simulink model "Controller_Algorithm_Local"  (R2025b)
settings: Solver=FixedStepAuto  StartTime=0.0  StopTime=10.0  RelTol=1e-3
InitFcn:
  | Simulink.defineIntEnumType(...
  | 'modeSchedulerEnum', ...
  | {'Error', 'OpenLoopVelocity', 'CalibrateEncoder', 'Velocity'}, ...
  | [0, 1, 2, 3]);
values from neighbouring files (symbols this model uses):
  sampleTime = 4.0E-5    [FoCFpgaData.sldd]
settings Model: DataDictionary=FoCFpgaData.sldd  Creator=Admin  LastModifiedBy=Admin
settings SolverCC: ZeroCrossAlgorithm=Adaptive
settings DataIOCC: LimitDataPoints=on  SaveFormat=Structure  SaveOutput=off  SaveTime=off
settings OptimizationCC: DefaultParameterBehavior=Inlined  UseDivisionForNetSlopeComputation=on
settings ConfigComp: CovMetricSettings=dw  CovSaveCumulativeToWorkspaceVar=on  CovSaveSingleToWorkspaceVar=on  CovExternalEMLEnable=off  CovSFcnEnable=off

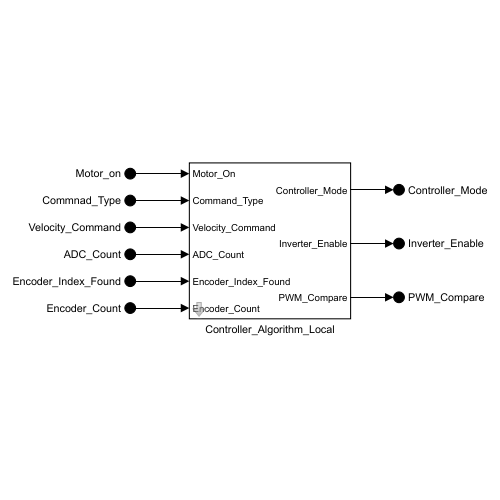
[thumbnail: Simulink's stored preview of the top-level diagram]
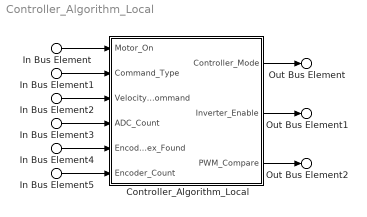
== system Controller_Algorithm_Local ==
  In Bus Element : Inport  PortName=Motor_on
  In Bus Element1 : Inport  Port=2  PortName=Commnad_Type
  In Bus Element2 : Inport  Port=3  PortName=Velocity_Command
  In Bus Element3 : Inport  Port=4  PortName=ADC_Count
  In Bus Element4 : Inport  Port=5  PortName=Encoder_Index_Found
  In Bus Element5 : Inport  Port=6  PortName=Encoder_Count
  Controller_Algorithm_Local : Subsystem
      mask help: Simulink:masks:GenSFuncDesc_MD
      mask Help: eval('feval(''rtwprivate'',''rtwhelpview'',''rtw_sfcn_block'')');
  Out Bus Element : Outport  PortName=Controller_Mode
  Out Bus Element1 : Outport  Port=2  PortName=Inverter_Enable
  Out Bus Element2 : Outport  Port=3  PortName=PWM_Compare
  wires:
  In Bus Element4/1 -> Controller_Algorithm_Local/5(Encoder_Index_Found)
  In Bus Element5/1 -> Controller_Algorithm_Local/6(Encoder_Count)
  Controller_Algorithm_Local/1(Controller_Mode) -> Out Bus Element/1
  Controller_Algorithm_Local/2(Inverter_Enable) -> Out Bus Element1/1
  Controller_Algorithm_Local/3(PWM_Compare) -> Out Bus Element2/1
  In Bus Element/1 -> Controller_Algorithm_Local/1(Motor_On)
  In Bus Element1/1 -> Controller_Algorithm_Local/2(Command_Type)
  In Bus Element2/1 -> Controller_Algorithm_Local/3(Velocity_Command)
  In Bus Element3/1 -> Controller_Algorithm_Local/4(ADC_Count)

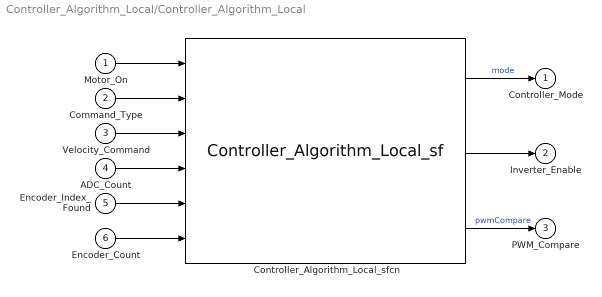
== system Controller_Algorithm_Local/Controller_Algorithm_Local ==
  Motor_On : Inport  SampleTime=sampleTime.VelocityControl  Interpolate=off
  Command_Type : Inport  Port=2  Interpolate=off
  Velocity_Command : Inport  Port=3
  ADC_Count : Inport  Port=4  PortDimensions=2  SampleTime=sampleTime.CurrentControl  Interpolate=off
  Encoder_Index_Found : Inport  Port=5  Interpolate=off
  Encoder_Count : Inport  Port=6  Interpolate=off
  Controller_Algorithm_Local_sfcn : S-Function  FunctionName=Controller_Algorithm_Local_sf  SFunctionModules=""  SFunctionDeploymentMode=off  EnableBusSupport=off  SFcnStateName=DWORK0,DWORK1,DWORK2,DWORK3,DWORK4,DWORK5,DWORK6,DWORK7,DWORK8,DWORK9,DWORK15,DWORK16,DWORK17,DWORK18,DWORK19,DWORK20,DWORK21,DWORK22,DWORK23,DWORK24,DWORK25,DWORK26,DWORK27,DWORK28,DWORK29,DWORK30,DWORK31,DWORK32,DWORK33,DWORK34,DWORK35,DWORK37,DWORK38,DWORK39,DWORK40,DWORK41,DWORK42,DWORK43,DWORK44,DWORK45,DWORK46,DWORK47,DWORK48,DWORK49  mask{rtw_sf_name=Controller_Algorithm_Local_sf, showVar=off}
      mask prompts: rtw_sf_name "Simulink:masks:GenSFuncName_MP"; showVar "Simulink:masks:GenSFuncShowModuleList_MP"
      mask help: Simulink:masks:GenSFuncDesc_MD
      mask init:
      | displist = '';
      | if ~strcmp(get_param(gcb, 'FunctionName'), rtw_sf_name);
      |   set_param(gcb, 'FunctionName', rtw_sf_name);
      | end
      | % Check if we are generating code
      | rtw_mode = false;
      | if strcmpi(get_param(bdroot(gcb),'SimulationStatus'),'Initializing')
      | 	rtw_mode = strcmpi(get_param(bdroot(gcb),'BuildingRTWCode'),'on') && ...
      | 		~strcmpi(get_param(bdroot(gcb),'TargetStyle'),'SimulationTarget');
      | end
      | if showVar || rtw_mode
      | 	if exist('rtwsfunc') == 2 | exist('rtwsfunc') == 6
      | 		tmplist = rtwsfunc(rtw_sf_name,gcb);
      | 		tmplist = DAStudio.message('Simulink:masks:GenSFuncListOfModules_IC', tmplist);
      | 	elseif showVar
      | 		tmplist1 = DAStudio.message('Simulink:masks:GenSFuncListOfModules_IC', '');
      |         tmplist2 = DAStudio.message('Simulink:masks:GenSFuncNotLicensed_IC');
      |         tmplist = [tmplist1 tmplist2];
      |  	end
      | end
      | if showVar
      |   displist = tmplist;
      | end
      settings: SFcnIsStateOwnerBlock=on
      settings: CopyFcn=|
      | if ~strcmp(get_param(gcb,'Linkstatus'),'none') && ...
      | ~strcmp(get_param(gcb,'Linkstatus'),'implicit')
      |   set_param(gcb,'LinkStatus','none');
      | end
      mask Help: eval('feval(''rtwprivate'',''rtwhelpview'',''rtw_sfcn_block'')');
      mask Display:
      | port_label('input',1,'Motor_On');
      | port_label('input',2,'Command_Type');
      | port_label('input',3,'Velocity_Command');
      | port_label('input',4,'ADC_Count');
      | port_label('input',5,'Encoder_Index_Found');
      | port_label('input',6,'Encoder_Count');
      | port_label('output',1,'Controller_Mode');
      | port_label('output',2,'Inverter_Enable');
      | port_label('output',3,'PWM_Compare');
  Controller_Mode : Outport
  Inverter_Enable : Outport  Port=2
  PWM_Compare : Outport  Port=3
  wires:
  Motor_On/1 -> Controller_Algorithm_Local_sfcn/1
  Command_Type/1 -> Controller_Algorithm_Local_sfcn/2
  Velocity_Command/1 -> Controller_Algorithm_Local_sfcn/3
  ADC_Count/1 -> Controller_Algorithm_Local_sfcn/4
  Encoder_Index_Found/1 -> Controller_Algorithm_Local_sfcn/5
  Encoder_Count/1 -> Controller_Algorithm_Local_sfcn/6
  Controller_Algorithm_Local_sfcn/2 -> Inverter_Enable/1
  Controller_Algorithm_Local_sfcn/3 -> PWM_Compare/1  "pwmCompare"
  Controller_Algorithm_Local_sfcn/1 -> Controller_Mode/1  "mode"
